simulink model "LCK"  (R2018b)
settings: Solver=FixedStepDiscrete  StartTime=0.0  StopTime=inf  FixedStep=0.01  RelTol=1e-3
PostLoadFcn:
  | if any(exist('dsrtsu_mdlpostloadfcn', 'file') ~= 0), dsrtsu_mdlpostloadfcn('Execute', bdroot); end
values from neighbouring files (symbols this model uses):
  C_DEG2RAD = 0.0175    [LCK_Macro.sldd]
  C_KPH2MPS = 0.2778    [LCK_Macro.sldd]
  C_NEARZERO = 0.0001    [LCK_Macro.sldd]
  C_ONE = 1.0    [LCK_Macro.sldd]
  C_RAD2DEG = 57.2958    [LCK_Macro.sldd]
  C_ZERO = 0.0    [LCK_Macro.sldd]
  k_accel_pedal_pos_per_speed_x : value not decoded    [LCK_LogicPara.sldd]
  k_accel_pedal_pos_per_speed_z : value not decoded    [LCK_LogicPara.sldd]
  k_brake_suprress_hold = 1000.0    [LCK_LogicPara.sldd]
  k_driver_appl_torque_filt = 50.0    [LCK_LogicPara.sldd]
  k_driver_suppression_hold_time = 3000.0    [LCK_LogicPara.sldd]
  k_hands_on_wheel_hold_msec = 500.0    [LCK_LogicPara.sldd]
  k_hands_on_wheel_torque_hi = 0.2    [LCK_LogicPara.sldd]
  k_hands_on_wheel_torque_lo = 0.15    [LCK_LogicPara.sldd]
  k_handsoff_delay_cycles = 50.0    [LCK_LogicPara.sldd]
  k_handsoff_torq_Lo_CR = 0.3    [LCK_LogicPara.sldd]
  k_handson_delay_cycles = 5.0    [LCK_LogicPara.sldd]
  k_HighAccel_suppress_hold = 3000.0    [LCK_LogicPara.sldd]
  k_HLR_suprress_hold = 3000.0    [LCK_LogicPara.sldd]
  k_hs_StrAng_CR_threshold_z : value not decoded    [LCK_LogicPara.sldd]
  k_LC_Exit_Switch = 0.0    [LCK_LogicPara.sldd]
  k_LCG_Configured = 1.0    [LCK_LogicPara.sldd]
  k_LCK_A0_Rdy2Act_UseConst = 0.0    [LCK_LogicPara.sldd]
  k_LCK_A0Fac_ActSta : value not decoded    [LCK_CtrlPara.sldd]
  k_LCK_A0Fac_DrvStm : value not decoded    [LCK_CtrlPara.sldd]
  k_LCK_A0Shift_LftCurv : value not decoded    [LCK_CtrlPara.sldd]
  k_LCK_A0Shift_RgtCurv : value not decoded    [LCK_CtrlPara.sldd]
  k_LCK_A0Shift_StraLan = 0.0    [LCK_CtrlPara.sldd]
  k_LCK_A0ShiftFac_Dy_LftCurv : value not decoded    [LCK_CtrlPara.sldd]
  k_LCK_A0ShiftFac_Dy_RgtCurv : value not decoded    [LCK_CtrlPara.sldd]
  k_LCK_A0ShiftFac_Vspd : value not decoded    [LCK_CtrlPara.sldd]
  k_LCK_accel_inhibit_thold = 35.0    [LCK_LogicPara.sldd]
  k_LCK_Active2Ready_Mask = 255.0    [LCK_LogicPara.sldd]
  k_LCK_CvatRateBks : value not decoded    [LCK_CtrlPara.sldd]
  k_LCK_CvatrBks : value not decoded    [LCK_CtrlPara.sldd]
  k_LCK_DFac_Dy : value not decoded    [LCK_CtrlPara.sldd]
  k_LCK_DFac_Dy_Curv : value not decoded    [LCK_CtrlPara.sldd]
  k_LCK_DFac_HaCurCen : value not decoded    [LCK_CtrlPara.sldd]
  k_LCK_DFac_HaCurSid : value not decoded    [LCK_CtrlPara.sldd]
  k_LCK_DFac_HadCurCen : value not decoded    [LCK_CtrlPara.sldd]
  k_LCK_DFac_HadCurSid : value not decoded    [LCK_CtrlPara.sldd]
  k_LCK_DFac_HadStrCen : value not decoded    [LCK_CtrlPara.sldd]
  k_LCK_DFac_HadStrSid : value not decoded    [LCK_CtrlPara.sldd]
  k_LCK_DFac_HaStrCen : value not decoded    [LCK_CtrlPara.sldd]
  k_LCK_DFac_HaStrSid : value not decoded    [LCK_CtrlPara.sldd]
  k_LCK_DFac_Rad : value not decoded    [LCK_CtrlPara.sldd]
  k_LCK_DFac_SA_CurCen : value not decoded    [LCK_CtrlPara.sldd]
  k_LCK_DFac_SA_CurSid : value not decoded    [LCK_CtrlPara.sldd]
  k_LCK_DFac_SA_StrCen : value not decoded    [LCK_CtrlPara.sldd]
  k_LCK_DFac_SA_StrSid : value not decoded    [LCK_CtrlPara.sldd]
  k_LCK_DFac_SS_CurCen : value not decoded    [LCK_CtrlPara.sldd]
  k_LCK_DFac_SS_CurSid : value not decoded    [LCK_CtrlPara.sldd]
  k_LCK_DFac_SS_StrCen : value not decoded    [LCK_CtrlPara.sldd]
  k_LCK_DFac_SS_StrSid : value not decoded    [LCK_CtrlPara.sldd]
  k_LCK_DFac_Vspd : value not decoded    [LCK_CtrlPara.sldd]
  k_LCK_DlyTm_DrvStim = 0.2    [LCK_CtrlPara.sldd]
  k_LCK_DTermMax = 2.0    [LCK_CtrlPara.sldd]
  k_LCK_DyBks_Curv : value not decoded    [LCK_CtrlPara.sldd]
  k_LCK_Enable_POOnly = 1.0    [LCK_LogicPara.sldd]
  k_LCK_Entry_DistBuffer = 0.1    [LCK_LogicPara.sldd]
  k_LCK_Fac_Vspd2RngThr_FalRec = 0.23    [LCK_CtrlPara.sldd]
  k_LCK_Ffw_CvatSwh = 0.0    [LCK_CtrlPara.sldd]
  k_LCK_Ffw_DyBks : value not decoded    [LCK_CtrlPara.sldd]
  k_LCK_Ffw_TimCon_CmdFlt = 0.0    [LCK_CtrlPara.sldd]
  k_LCK_FfwDeltaFac_Rad_Lft : value not decoded    [LCK_CtrlPara.sldd]
  k_LCK_FfwDeltaFac_Rad_Rgt : value not decoded    [LCK_CtrlPara.sldd]
  k_LCK_FfwDeltaFac_Vspd : value not decoded    [LCK_CtrlPara.sldd]
  k_LCK_FfwFac_CvatRate_Lft : value not decoded    [LCK_CtrlPara.sldd]
  k_LCK_FfwFac_CvatRate_Rgt : value not decoded    [LCK_CtrlPara.sldd]
  k_LCK_FfwFac_Dy : value not decoded    [LCK_CtrlPara.sldd]
  k_LCK_FfwFac_Rad_Lft : value not decoded    [LCK_CtrlPara.sldd]
  k_LCK_FfwFac_Rad_Rgt : value not decoded    [LCK_CtrlPara.sldd]
  k_LCK_FfwFac_Vspd : value not decoded    [LCK_CtrlPara.sldd]
  k_LCK_FfwTorq_Cvat : value not decoded    [LCK_CtrlPara.sldd]
  k_LCK_HAFac_ActSta : value not decoded    [LCK_CtrlPara.sldd]
  k_LCK_HAFac_DrvStm : value not decoded    [LCK_CtrlPara.sldd]
  k_LCK_HaloTime = 2000.0    [LCK_LogicPara.sldd]
  k_LCK_HaloTime_Switch = 0.0    [LCK_LogicPara.sldd]
  k_LCK_HARFac_ActSta : value not decoded    [LCK_CtrlPara.sldd]
  k_LCK_HARFac_DrvStm : value not decoded    [LCK_CtrlPara.sldd]
  k_LCK_Hed_DyBks : value not decoded    [LCK_CtrlPara.sldd]
  k_LCK_HedAngDiffX : value not decoded    [LCK_CtrlPara.sldd]
  k_LCK_HedAngRateDiffX : value not decoded    [LCK_CtrlPara.sldd]
  k_LCK_HndsOnWhel_DlyTm_Idl2Rdy = 0.0    [LCK_LogicPara.sldd]
  k_LCK_host_veh_width = 1.86    [LCK_LogicPara.sldd]
  k_LCK_Idle2Ready_Mask = 239.0    [LCK_LogicPara.sldd]
  k_LCK_Junc_SusTime = 1.0    [LCK_LogicPara.sldd]
  k_LCK_KpKdDecSlopeLmt = 10.0    [LCK_CtrlPara.sldd]
  k_LCK_KpKdIncSlopeLmt = 5.0    [LCK_CtrlPara.sldd]
  k_LCK_Lat_Ctrl_DFac_Lft = 1.0    [LCK_CtrlPara.sldd]
  k_LCK_Lat_Ctrl_DFac_Rgt = 1.05    [LCK_CtrlPara.sldd]
  k_LCK_Lat_Ctrl_Kd = 0.8    [LCK_CtrlPara.sldd]
  k_LCK_Lat_Ctrl_Ki = 0.5    [LCK_CtrlPara.sldd]
  k_LCK_Lat_Ctrl_Kp = 0.7    [LCK_CtrlPara.sldd]
  k_LCK_Lat_Ctrl_Kp_NearGain = 0.7    [LCK_CtrlPara.sldd]
  k_LCK_Lat_Ctrl_PFac_Lft = 1.0    [LCK_CtrlPara.sldd]
  k_LCK_Lat_Ctrl_PFac_Rgt = 1.05    [LCK_CtrlPara.sldd]
  k_LCK_Lat_Ctrl_TimCon_CmdFlt = 5.0    [LCK_CtrlPara.sldd]
  k_LCK_Lat_DFac_Rad : value not decoded    [LCK_CtrlPara.sldd]
  k_LCK_Lat_DFac_SS_Cur : value not decoded    [LCK_CtrlPara.sldd]
  k_LCK_Lat_DFac_SS_Str : value not decoded    [LCK_CtrlPara.sldd]
  k_LCK_Lat_DFac_Vspd : value not decoded    [LCK_CtrlPara.sldd]
  k_LCK_Lat_DyBks : value not decoded    [LCK_CtrlPara.sldd]
  k_LCK_Lat_IFac_Rad : value not decoded    [LCK_CtrlPara.sldd]
  k_LCK_Lat_IFac_Vspd : value not decoded    [LCK_CtrlPara.sldd]
  k_LCK_Lat_ILmtFac_Dy_CurvLan : value not decoded    [LCK_CtrlPara.sldd]
  k_LCK_Lat_ILmtFac_Dy_StraLan : value not decoded    [LCK_CtrlPara.sldd]
  k_LCK_Lat_ILmtFac_Rad : value not decoded    [LCK_CtrlPara.sldd]
  k_LCK_Lat_ILmtFac_Rad_NearGain = 1.0    [LCK_CtrlPara.sldd]
  k_LCK_Lat_ILmtFac_Vspd_CurvLan : value not decoded    [LCK_CtrlPara.sldd]
  k_LCK_Lat_ILmtFac_Vspd_StraLan : value not decoded    [LCK_CtrlPara.sldd]
  k_LCK_Lat_ITermLmt_Dy = 1.0    [LCK_CtrlPara.sldd]
  k_LCK_Lat_KpKdDecSlopeLmt = 10.0    [LCK_CtrlPara.sldd]
  k_LCK_Lat_KpKdIncSlopeLmt = 10.0    [LCK_CtrlPara.sldd]
  k_LCK_Lat_PFac_Dy_InnLftCur : value not decoded    [LCK_CtrlPara.sldd]
  k_LCK_Lat_PFac_Dy_InnRgtCur : value not decoded    [LCK_CtrlPara.sldd]
  k_LCK_Lat_PFac_Dy_OutLftCur : value not decoded    [LCK_CtrlPara.sldd]
  k_LCK_Lat_PFac_Dy_OutRgtCur : value not decoded    [LCK_CtrlPara.sldd]
  k_LCK_Lat_PFac_Dy_Str : value not decoded    [LCK_CtrlPara.sldd]
  k_LCK_Lat_PFac_Rad : value not decoded    [LCK_CtrlPara.sldd]
  ... (+153 more)
undefined symbols (not defined in the file or in its folder): k_LCK_CurvBks, K_LCK_SPA0A1A2_LMRngCmp_y
libraries: LateralControl_fcns_lib x59, simulink x24
(part 19 of 47)

== system LCK/Lateral_Control_Module/Adas_Lateral_Control_LCK_Core/Module 3/Sig_Wekng_0 ==
  Lat_Ctrl_State : Inport
  Constant3 : Constant  Tag={'output',{'type','Int32'},'date',737462.5090449769}  Description=_GWMH9P4.LCK.000_208_
  Constant4 : Constant  Tag={'output',{'type','Int32'},'date',737462.5090449769}  Description=_GWMH9P4.LCK.000_208_  Value=0
  Constant5 : Constant  Tag={'output',{'type','Int32'},'date',737462.5090449769}  Description=_GWMH9P4.LCK.000_208_  OutDataTypeStr=single
  Constant6 : Constant  Tag={'output',{'type','Int32'},'date',737462.5090449769}  Description=_GWMH9P4.LCK.000_208_  OutDataTypeStr=single
  Constant7 : Constant  Tag={'output',{'type','Int32'},'date',737462.5090449769}  Description=_GWMH9P4.LCK.000_208_  OutDataTypeStr=single
  Data Type Conversion54 : DataTypeConversion  Description=_GACA26P4.LCK.000_208_
  Logical Operator8 : Logic  Tag={'date',737531.60623578704}  Description=_GACA26P4.LCK.000_215_  AllPortsSameDT=off  OutDataTypeStr=boolean
  Relational Operator14 : RelationalOperator  Tag={'date',737531.60624731483}  Description=_GACA26P4.LCK.000_225_  Operator===  OutDataTypeStr=boolean  RndMeth=Nearest
  Relational Operator15 : RelationalOperator  Tag={'date',737531.60624776618}  Description=_GACA26P4.LCK.000_226_  Operator===  OutDataTypeStr=boolean  RndMeth=Nearest
  Switch3 : Switch  Tag={'output',{'type','Float32'},'threshold',{'type','Int32'},'date',737463.80838512734}  Description=_GWMH9P4.LCK.000_251_  Threshold=0.5
  Switch4 : Switch  Tag={'output',{'type','Float32'},'threshold',{'type','Int32'},'date',737463.80838512734}  Description=_GWMH9P4.LCK.000_251_  Threshold=0.5
  Switch5 : Switch  Tag={'output',{'type','Float32'},'threshold',{'type','Int32'},'date',737463.80838512734}  Description=_GWMH9P4.LCK.000_251_  Threshold=0.5
  Trigger Hold Counter : Subsystem
  Unit Delay2 : UnitDelay  Tag={'output',{'inheritscaling',1},'state',{'type','Int32'},'date',737531.81169192132}  Description=_GACA26P4.LCK.000_260_  SampleTime=-1
  k_LCK_A0Fac_ActSta : Lookup_n-D  Tag={'input',{'name','$P','class','EXTERN_CAL','type','Float32'},'output',{'type','Float32'},'table',{'name','$P','class','EXTERN_CAL','type','Float32'},'date',737534.7265986806}  NumberOfTableDimensions=1  BreakpointsForDimension1=k_LCK_TimBks_ActSta  IndexSearchMethod=Linear search  Table=k_LCK_A0Fac_ActSta  ExtrapMethod=Clip  InternalRulePriority=Speed  RndMeth=Simplest  InputSameDT=on
  k_LCK_HAFac_ActSta : Lookup_n-D  Tag={'input',{'name','$P','class','EXTERN_CAL','type','Float32'},'output',{'type','Float32'},'table',{'name','$P','class','EXTERN_CAL','type','Float32'},'date',737534.7265986806}  NumberOfTableDimensions=1  BreakpointsForDimension1=k_LCK_TimBks_ActSta  IndexSearchMethod=Linear search  Table=k_LCK_HAFac_ActSta  ExtrapMethod=Clip  InternalRulePriority=Speed  RndMeth=Simplest  InputSameDT=on
  k_LCK_HARFac_ActSta : Lookup_n-D  Tag={'input',{'name','$P','class','EXTERN_CAL','type','Float32'},'output',{'type','Float32'},'table',{'name','$P','class','EXTERN_CAL','type','Float32'},'date',737534.7265986806}  NumberOfTableDimensions=1  BreakpointsForDimension1=k_LCK_TimBks_ActSta  IndexSearchMethod=Linear search  Table=k_LCK_HARFac_ActSta  ExtrapMethod=Clip  InternalRulePriority=Speed  RndMeth=Simplest  InputSameDT=on
  k_LCK_SigFacHldTim_ActSta : Constant  Tag={'output',{'name','$P','class','EXTERN_CAL','type','UInt16'},'date',737534.72887515044}  Description=_GACA26P4.LCK.000_264_  Value=k_LCK_SigFacHldTim_ActSta
  A0Fac_ActSta : Outport
  HAFac_ActSta : Outport  Port=2
  HARFac_ActSta : Outport  Port=3
  Act_Start_Falg_Held : Outport  Port=4
  wires:
  Logical Operator8/1 -> Data Type Conversion54/1
  Relational Operator14/1 -> Logical Operator8/2
  Relational Operator15/1 -> Logical Operator8/1
  Constant3/1 -> Relational Operator15/1
  Constant4/1 -> Relational Operator14/2
  Unit Delay2/1 -> Relational Operator14/1
  Lat_Ctrl_State/1 -> Unit Delay2/1, Relational Operator15/2
  Data Type Conversion54/1 -> Trigger Hold Counter/1(Trigger)
  Trigger Hold Counter/1(Out) -> Act_Start_Falg_Held/1, Switch5/2, Switch4/2, Switch3/2
  Switch4/1 -> A0Fac_ActSta/1
  Constant7/1 -> Switch4/3
  Constant5/1 -> Switch3/3
  Constant6/1 -> Switch5/3
  Switch3/1 -> HAFac_ActSta/1
  Switch5/1 -> HARFac_ActSta/1
  k_LCK_HARFac_ActSta/1 -> Switch5/1
  k_LCK_HAFac_ActSta/1 -> Switch3/1
  k_LCK_A0Fac_ActSta/1 -> Switch4/1
  Trigger Hold Counter/2(Counter) -> k_LCK_HARFac_ActSta/1, k_LCK_A0Fac_ActSta/1, k_LCK_HAFac_ActSta/1
  k_LCK_SigFacHldTim_ActSta/1 -> Trigger Hold Counter/2(hold_time)
